simulink model "Simulation_Model"  (R2023b)
settings: Solver=daessc  StartTime=0.0  StopTime=45  RelTol=1e-3
undefined symbols (not defined in the file): t_sample
libraries: Simulation_lib x1, SignalEditorBlockLib x1
settings Model: Creator=FIRSTMentor  LastModifiedBy=ander
settings DebuggingCC: UnderspecifiedInitializationDetection=Classic  MergeDetectMultiDrivingBlocksExec=none
settings ModelReferenceCC: PropagateSignalLabelsOutOfModel=off

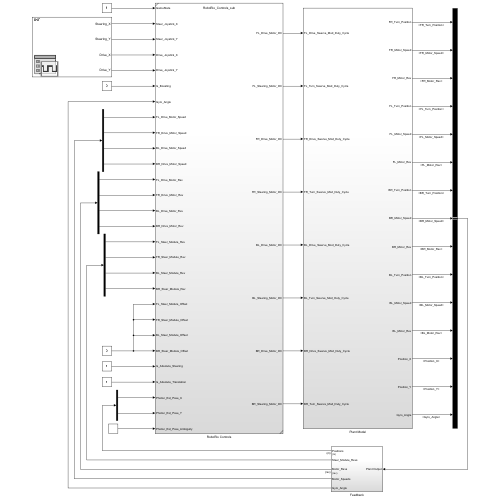
[thumbnail: Simulink's stored preview of the top-level diagram]
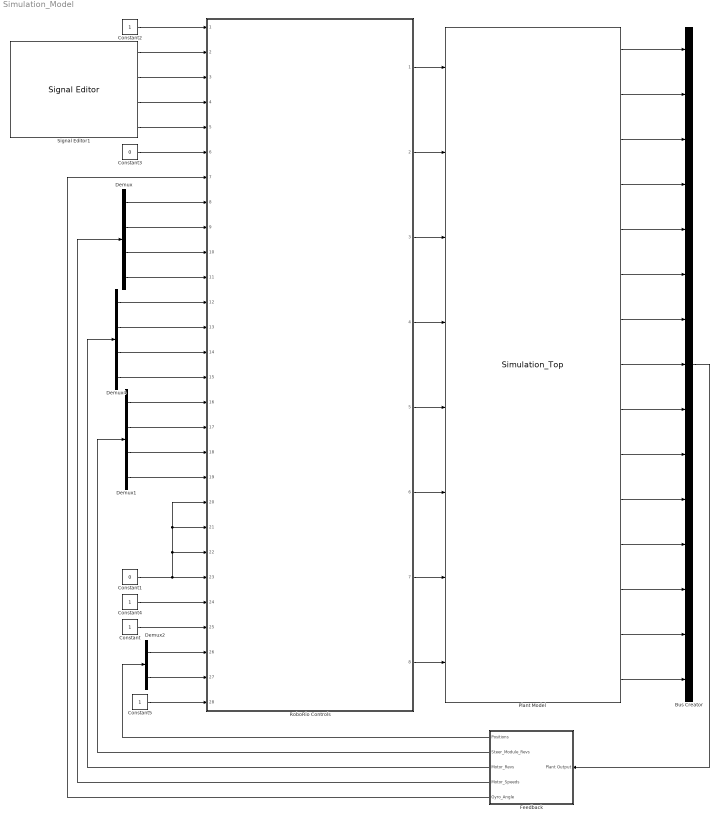
== system Simulation_Model ==
  Bus Creator : BusCreator  Inputs=15
  Constant : Constant  OutDataTypeStr=boolean
  Constant1 : Constant  Value=0
  Constant2 : Constant
  Constant3 : Constant  Value=0  OutDataTypeStr=boolean
  Constant4 : Constant  OutDataTypeStr=boolean
  Constant5 : Constant  OutDataTypeStr=double
  Demux : Demux
  Demux1 : Demux
  Demux2 : Demux  Outputs=2
  Demux4 : Demux
  Feedback : Subsystem
  Plant Model : Simulation_lib/Simulation_Top  SystemSampleTime=-1  VariantActivationTime=update diagram  AllowFlexibleInterface=on  Latency=0  AutoFrameSizeCalculation=off
  RoboRio Controls : Subsystem  ReferencedSubsystem=RoboRio_Controls_sub
  Signal Editor1 : SignalEditorBlockLib/Signal Editor  FileName=Joystick_input_test_data.mat  ActiveScenario=DXP  ActiveSignal=Drive_Y  IsBus=off  OutputBusObjectStr=Bus: BusObject  SampleTime=t_sample  ZeroCross=off  OutputAfterFinalValue=Setting to zero  Unit=inherit  PreserveSignalName=on  ApplySigPropsToAllScenarios=on  ApplySigPropsToAllSignals=off
  wires:
  RoboRio Controls/3 -> Plant Model/3
  RoboRio Controls/2 -> Plant Model/2
  RoboRio Controls/4 -> Plant Model/4
  RoboRio Controls/1 -> Plant Model/1
  RoboRio Controls/5 -> Plant Model/5
  RoboRio Controls/6 -> Plant Model/6
  RoboRio Controls/7 -> Plant Model/7
  RoboRio Controls/8 -> Plant Model/8
  Constant/1 -> RoboRio Controls/25
  Constant1/1 -> RoboRio Controls/20, RoboRio Controls/21, RoboRio Controls/22, RoboRio Controls/23
  Constant2/1 -> RoboRio Controls/1
  Signal Editor1/2 -> RoboRio Controls/3
  Signal Editor1/4 -> RoboRio Controls/5
  Constant3/1 -> RoboRio Controls/6
  Signal Editor1/3 -> RoboRio Controls/4
  Signal Editor1/1 -> RoboRio Controls/2
  Constant4/1 -> RoboRio Controls/24
  Plant Model/7 -> Bus Creator/7
  Plant Model/6 -> Bus Creator/6
  Plant Model/8 -> Bus Creator/8
  Plant Model/5 -> Bus Creator/5
  Plant Model/9 -> Bus Creator/9
  Plant Model/4 -> Bus Creator/4
  Plant Model/10 -> Bus Creator/10
  Plant Model/3 -> Bus Creator/3
  Plant Model/11 -> Bus Creator/11
  Plant Model/2 -> Bus Creator/2
  Plant Model/12 -> Bus Creator/12
  Plant Model/1 -> Bus Creator/1
  Plant Model/13 -> Bus Creator/13
  Bus Creator/1 -> Feedback/1(Plant Output)
  Feedback/4(Motor_Speeds) -> Demux/1
  Demux/2 -> RoboRio Controls/9
  Demux/1 -> RoboRio Controls/8
  Demux/3 -> RoboRio Controls/10
  Demux/4 -> RoboRio Controls/11
  Demux1/1 -> RoboRio Controls/16
  Demux1/2 -> RoboRio Controls/17
  Demux1/3 -> RoboRio Controls/18
  Demux1/4 -> RoboRio Controls/19
  Feedback/2(Steer_Module_Revs) -> Demux1/1
  Feedback/5(Gyro_Angle) -> RoboRio Controls/7
  Demux4/1 -> RoboRio Controls/12
  Demux4/2 -> RoboRio Controls/13
  Demux4/3 -> RoboRio Controls/14
  Demux4/4 -> RoboRio Controls/15
  Feedback/3(Motor_Revs) -> Demux4/1
  Plant Model/14 -> Bus Creator/14
  Plant Model/15 -> Bus Creator/15
  Demux2/2 -> RoboRio Controls/27
  Demux2/1 -> RoboRio Controls/26
  Feedback/1(Positions) -> Demux2/1
  Constant5/1 -> RoboRio Controls/28

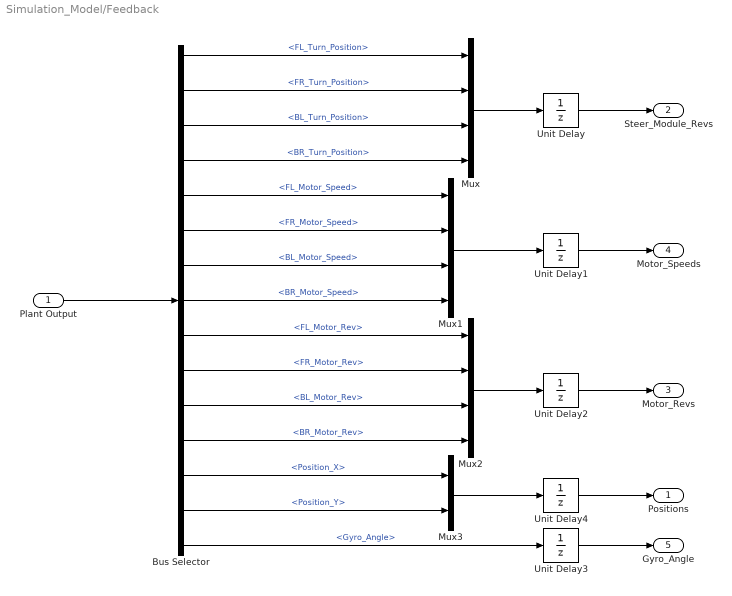
== system Simulation_Model/Feedback ==
  Plant Output : Inport
  Bus Selector : BusSelector  OutputSignals=FL_Turn_Position,FR_Turn_Position,BL_Turn_Position,BR_Turn_Position,FL_Motor_Speed,FR_Motor_Speed,BL_Motor_Speed,BR_Motor_Speed,FL_Motor_Rev,FR_Motor_Rev,BL_Motor_Rev,BR_Motor_Rev,Position_X,Position_Y,Gyro_Angle
  Mux : Mux
  Mux1 : Mux
  Mux2 : Mux
  Mux3 : Mux  Inputs=2
  Unit Delay : UnitDelay  InitialCondition=[0 0 0 0]  SampleTime=t_sample  HasFrameUpgradeWarning=on
  Unit Delay1 : UnitDelay  InitialCondition=[0 0 0 0]  SampleTime=t_sample  HasFrameUpgradeWarning=on
  Unit Delay2 : UnitDelay  InitialCondition=[0 0 0 0]  SampleTime=t_sample  HasFrameUpgradeWarning=on
  Unit Delay3 : UnitDelay  SampleTime=t_sample  HasFrameUpgradeWarning=on
  Unit Delay4 : UnitDelay  SampleTime=t_sample  HasFrameUpgradeWarning=on
  Positions : Outport  Unit=m
  Steer_Module_Revs : Outport  Port=2
  Motor_Revs : Outport  Port=3  Unit=rev
  Motor_Speeds : Outport  Port=4
  Gyro_Angle : Outport  Port=5
  wires:
  Plant Output/1 -> Bus Selector/1
  Mux/1 -> Unit Delay/1
  Mux1/1 -> Unit Delay1/1
  Mux2/1 -> Unit Delay2/1
  Bus Selector/15 -> Unit Delay3/1  "<Gyro_Angle>"
  Bus Selector/1 -> Mux/1  "<FL_Turn_Position>"
  Bus Selector/2 -> Mux/2  "<FR_Turn_Position>"
  Bus Selector/3 -> Mux/3  "<BL_Turn_Position>"
  Bus Selector/4 -> Mux/4  "<BR_Turn_Position>"
  Bus Selector/5 -> Mux1/1  "<FL_Motor_Speed>"
  Bus Selector/6 -> Mux1/2  "<FR_Motor_Speed>"
  Bus Selector/7 -> Mux1/3  "<BL_Motor_Speed>"
  Bus Selector/8 -> Mux1/4  "<BR_Motor_Speed>"
  Bus Selector/9 -> Mux2/1  "<FL_Motor_Rev>"
  Bus Selector/10 -> Mux2/2  "<FR_Motor_Rev>"
  Bus Selector/11 -> Mux2/3  "<BL_Motor_Rev>"
  Bus Selector/12 -> Mux2/4  "<BR_Motor_Rev>"
  Unit Delay/1 -> Steer_Module_Revs/1
  Unit Delay1/1 -> Motor_Speeds/1
  Unit Delay2/1 -> Motor_Revs/1
  Unit Delay3/1 -> Gyro_Angle/1
  Bus Selector/13 -> Mux3/1  "<Position_X>"
  Bus Selector/14 -> Mux3/2  "<Position_Y>"
  Mux3/1 -> Unit Delay4/1
  Unit Delay4/1 -> Positions/1
